simulink model "mm_autograde_M2_nice"  (R2025a)
settings: Solver=FixedStepAuto  StartTime=0.0  StopTime=500  FixedStep=0.005  RelTol=1e-3
libraries: mmuct_lib x1
settings Model: NumberOfSteps=20  SnapshotBufferSize=40  SnapshotInterval=20  Creator=nicolls  LastModifiedBy=llamalulu
settings RTWCC: GenCodeOnly=on

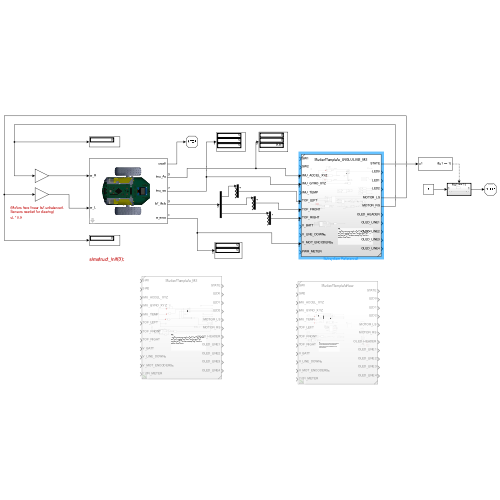
[thumbnail: Simulink's stored preview of the top-level diagram]
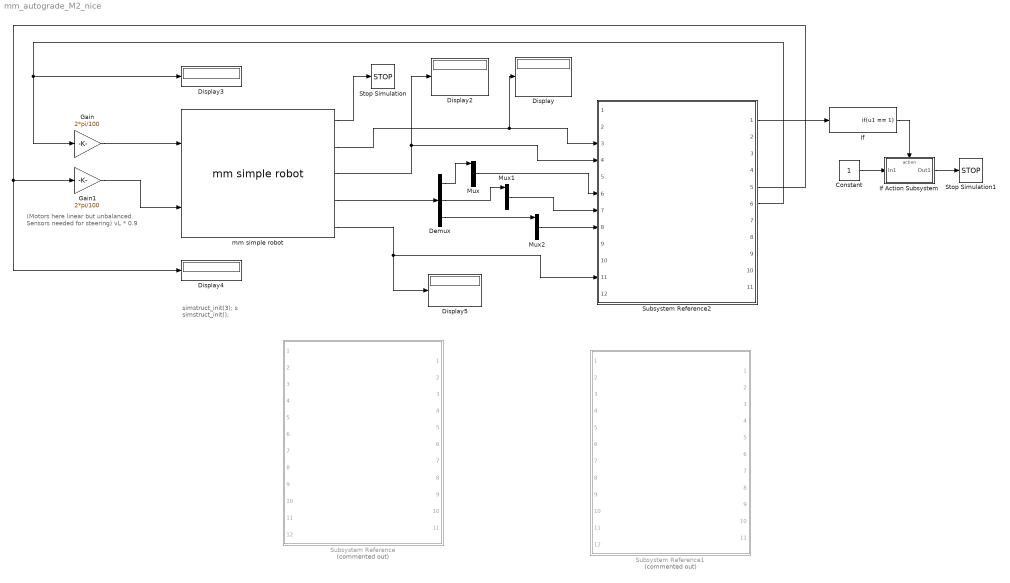
== system mm_autograde_M2_nice ==
  note: (Motors here linear but unbalanced.
      | Sensors needed for steering)
      |
      | vL * 0.9
  note: simstruct_init(3);
      | s
      | simstruct_init();
  Constant : Constant
  Demux : Demux  Outputs=3
  Display{,2..5} (5 alike) : Display
  Gain : Gain  Gain=2*pi/100
  Gain1 : Gain  Gain=2*pi/100
  If : If  IfExpression=u1 == 1  ShowElse=off  ZeroCross=off
  If Action Subsystem : Subsystem  TreatAsAtomicUnit=on
  Mux : Mux
  Mux1 : Mux
  Mux2 : Mux
  Stop Simulation : Stop
  Stop Simulation1 : Stop
  Subsystem Reference : Subsystem  Commented=on  ReferencedSubsystem=StudentTemplate_M2
  Subsystem Reference1 : Subsystem  Commented=on  ReferencedSubsystem=StudentTemplateNew
  Subsystem Reference2 : Subsystem  ReferencedSubsystem=StudentTemplate_LNGLUL002_M2
  mm simple robot : mmuct_lib/mm simple robot  simstruct=simstruct  x0=0.1  y0=0.1  theta0=0
      settings: SourceProductName=UCT EEE Micromouse
  wires:
  Demux/1 -> Mux/1
  Demux/2 -> Mux1/1
  Demux/3 -> Mux2/1
  mm simple robot/3 -> Subsystem Reference2/4, Display2/1
  mm simple robot/2 -> Subsystem Reference2/3, Display/1
  mm simple robot/5 -> Subsystem Reference2/11, Display5/1
  mm simple robot/4 -> Demux/1
  Gain1/1 -> mm simple robot/2
  Gain/1 -> mm simple robot/1
  mm simple robot/1 -> Stop Simulation/1
  Subsystem Reference2/1 -> If/1
  If Action Subsystem/1(Out1) -> Stop Simulation1/1
  If/1 -> If Action Subsystem/Action
  Constant/1 -> If Action Subsystem/1(In1)
  Subsystem Reference2/6 -> Gain/1, Display3/1
  Subsystem Reference2/5 -> Gain1/1, Display4/1
  Mux2/1 -> Subsystem Reference2/8
  Mux1/1 -> Subsystem Reference2/7
  Mux/1 -> Subsystem Reference2/6

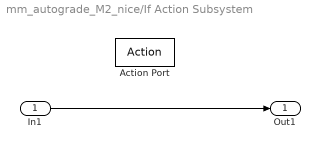
== system mm_autograde_M2_nice/If Action Subsystem ==
  In1 : Inport
  Action Port : ActionPort  ActionPortLabel=if(u1 == 1)
  Out1 : Outport
  wires:
  In1/1 -> Out1/1
